simulink model "st"  (R2022b)
settings: Solver=VariableStepAuto  StartTime=0.0  StopTime=1000  RelTol=1e-3
libraries: commsequence2 x2, commdigbbndpm3 x2, dspsrcs4 x2, commfilt2 x2, commchan3 x1, simulink x1, commsink2 x1, commsync2 x1, dspsigops x1
(part 1 of 2)
settings Model: Creator=svdvl  LastModifiedBy=svdvl

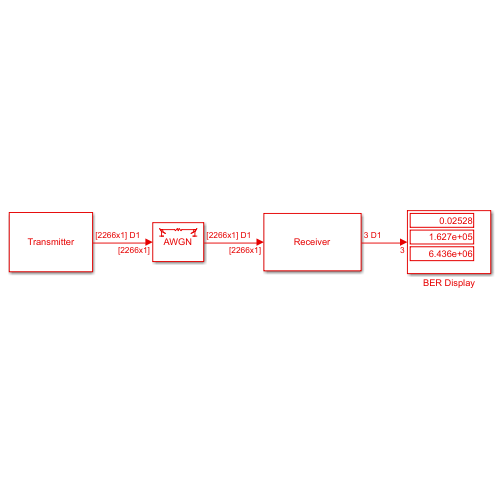
[thumbnail: Simulink's stored preview of the top-level diagram]
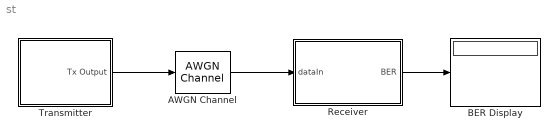
== system st ==
  AWGN Channel : commchan3/AWGN Channel  InputProcessing=Columns as channels (frame based)  seed=1  noiseMode="Signal to noise ratio  (Es/No)"  EbNodB=8  EsNodB=40  SNRdB=8  bitsPerSym=1  Ps=0.5  Tsym=2e-5  variance=1
  BER Display : Display
  Receiver : Subsystem
      mask Display: disp('Receiver')
  Transmitter : Subsystem
      mask Display: disp('Transmitter')
  wires:
  Transmitter/1(Tx Output) -> AWGN Channel/1
  AWGN Channel/1 -> Receiver/1(dataIn)
  Receiver/1(BER) -> BER Display/1

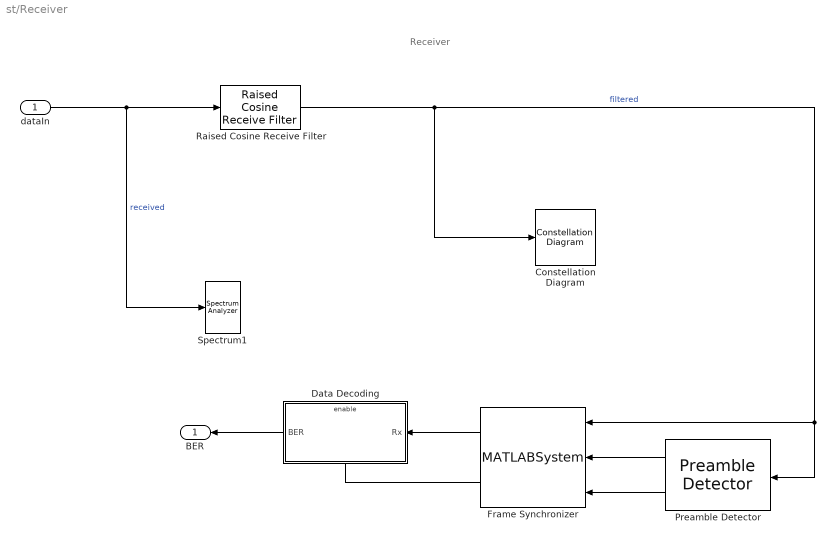
== system st/Receiver ==
  note: Receiver
  dataIn : Inport
  Constellation Diagram : ConstellationDiagram  WindowPosition=[-1346.000000,169.000000,600.000000,600.000000,]  Visible=on  ScopeFrameLocation=window  SamplesPerSymbol=1133  SymbolsToDisplaySource=Property  SymbolsToDisplay=1133  XLimits=[-1.46,1.46]  YLimits=[-1.38,1.38]  DefaultConfigurationName=comm.scopes.ConstellationDiagramBlockCfg
  Data Decoding : Subsystem
      mask Display: disp('Data Decoding');
  Frame Synchronizer : MATLABSystem  System=FrameSynchronizer  Input=Symbol  OutputFrameLength=1133  PreambleLength=13  SimulateUsing=Code generation
      mask Type: FrameSynchronizer
      mask Display:
      | disp(['Frame' char(10) 'Synchronizer']);
      | port_label('input',1,'u');
      | port_label('input',2,'idx');
      | port_label('input',3,'dtMt');
      | port_label('output',1,'Frame');
      | port_label('output',2,'Valid');
  Preamble Detector : commsync2/Preamble Detector  Input=Symbol  Preamble="sqrt(2)/2 * (-1-1i) * ([1     1     1     1     1    -1    -1     1     1    -1     1    -1     1])'"  Threshold=8  DetectionMetricOutput=on  Detections=First  SimulateUsing=Code generation
  Raised Cosine Receive Filter : commfilt2/Raised Cosine Receive Filter  filtType=Square root  R=0.5  filtSpan=12  N=2  downFactor=2  downOffset=0  filterGain=1  InputProcessing=Columns as channels (frame based)  RateOptions=Enforce single-rate processing  framing=Mute  checkCoeff=off  variableName=rcRxFilt  currentFiltSpan=10  D=5  inputOffset=0  sampMode=Mute  saveAsFlag=0  rateMode=Downsampling  checkGain=Normalized  launchFVT=on  roundingMode=Floor  overflowMode=off  coeffDataTypeStr=Inherit: Same word length as input  coeffMin=[]  coeffMax=[]  coeffLastDataTypeStr=Inherit: Same word length as input  accumDataTypeStr=Inherit: Same as product output  accumLastDataTypeStr=Inherit: Same as product output  outputDataTypeStr=Inherit: Same as accumulator  outputMin=[]  outputMax=[]  outputLastDataTypeStr=Inherit: Same as accumulator
  Spectrum1 : SpectrumAnalyzer
  BER : Outport  VectorParamsAs1DForOutWhenUnconnected=off
  wires:
  Raised Cosine Receive Filter/1 -> Constellation Diagram/1, Preamble Detector/1, Frame Synchronizer/1  "filtered"
  dataIn/1 -> Spectrum1/1, Raised Cosine Receive Filter/1  "received"
  Frame Synchronizer/1 -> Data Decoding/1(Rx)
  Preamble Detector/1 -> Frame Synchronizer/2
  Frame Synchronizer/2 -> Data Decoding/Enable
  Data Decoding/1(BER) -> BER/1
  Preamble Detector/2 -> Frame Synchronizer/3

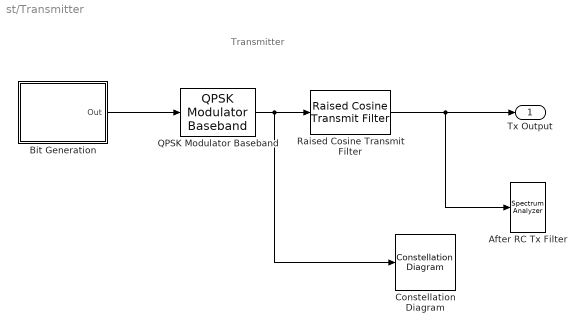
== system st/Transmitter ==
  note: Transmitter
  After RC Tx Filter : SpectrumAnalyzer
  Bit Generation : Subsystem
      mask Display: disp('Bits Generation')
  Constellation Diagram : ConstellationDiagram  WindowPosition=[-1247.000000,248.000000,600.000000,600.000000,]  Visible=on  ScopeFrameLocation=window  DefaultConfigurationName=comm.scopes.ConstellationDiagramBlockCfg
  QPSK Modulator Baseband : commdigbbndpm3/QPSK Modulator Baseband  InType=Bit  Enc=Gray  Ph=pi/4  outDtype=double  outWordLen=16  outUDDataType=sfix(16)  outFracLenMode=Best precision  outFracLen=15  outDataTypeStr=double  outLastDataTypeStr=double
  Raised Cosine Transmit Filter : commfilt2/Raised Cosine Transmit Filter  filtType=Square root  R=0.5  filtSpan=12  N=2  filterGain=1  InputProcessing=Columns as channels (frame based)  RateOptions=Enforce single-rate processing  framing=Mute  checkCoeff=off  variableName=rcTxFilt1  checkGain=Normalized  sampMode=Mute  saveAsFlag=0  currentFiltSpan=10  D=5  launchFVT=on  roundingMode=Floor  overflowMode=off  coeffDataTypeStr=Inherit: Same word length as input  coeffMin=[]  coeffMax=[]  coeffLastDataTypeStr=Inherit: Same word length as input  outputDataTypeStr=Inherit: Same as accumulator  outputMin=[]  outputMax=[]  outputLastDataTypeStr=Inherit: Same as accumulator
  Tx Output : Outport  VectorParamsAs1DForOutWhenUnconnected=off
  wires:
  Raised Cosine Transmit Filter/1 -> Tx Output/1, After RC Tx Filter/1
  Bit Generation/1(Out) -> QPSK Modulator Baseband/1
  QPSK Modulator Baseband/1 -> Constellation Diagram/1, Raised Cosine Transmit Filter/1

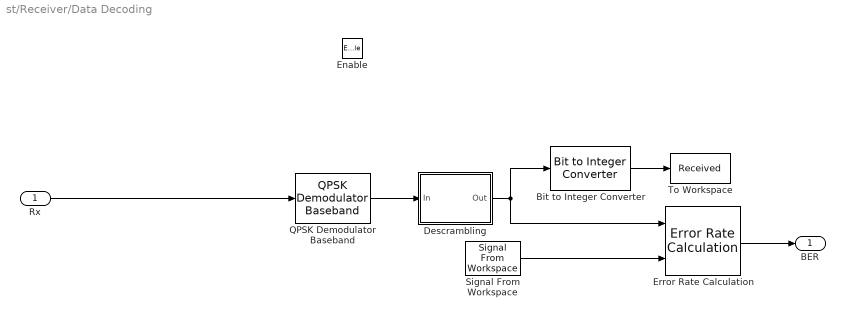
== system st/Receiver/Data Decoding ==
  Rx : Inport
  Enable : EnablePort
  Bit to Integer Converter : simulink/Logic and Bit Operations/Bit to Integer Converter  nbits=7  bitOrder=MSB first  signedOutputValues=Unsigned  outDtype=Inherit via internal rule  outDtypeSigned=Inherit via internal rule
      settings: LibrarySourceBlock=|
      | commutil2/Bit to Integer
      | Converter
  Descrambling : Subsystem
      mask Display: disp('Descrambling');
  Error Rate Calculation : commsink2/Error Rate Calculation  N=0  st_delay=0  cp_mode=Entire frame  subframe=ans.BerMask  PMode=Port  WsName=ErrorVec  RsMode2=off  stop=off  numErr=100  maxBits=1e6
  QPSK Demodulator Baseband : commdigbbndpm3/QPSK Demodulator Baseband  OutType=Bit  DecType=Hard decision  VarSource=Dialog  Variance=1  Dec=Gray  Ph=pi/4  outDtype1=Inherit via internal rule  outDtype2=Inherit via internal rule  derotateFactorWordLen=16  derotateFactorDataTypeStr=Inherit: Same word length as input  derotateFactorLastDataTypeStr=Inherit: Same word length as input
  Signal From Workspace : dspsrcs4/Signal From Workspace  X="[1\t0\t0\t1\t0\t0\t0\t1\t1\t0\t0\t1\t0\t1\t1\t1\t0\t1\t1\t0\t0\t1\t1\t0\t1\t1\t0\t0\t1\t1\t0\t1\t1\t1\t1\t0\t1\t0\t0\t0\t0\t0\t1\t1\t1\t0\t1\t1\t1\t1\t1\t0\t1\t1\t1\t1\t1\t1\t1\t0\t0\t1\t0\t1\t1\t0\t1\t1\t0\t0\t1\t1\t0\t0\t1\t0\t0\t0\t1\t0\t0\t0\t0\t0\t0\t1\t1\t0\t0\t0\t0\t0\t1\t1\t0\t0\t0\t0\t0\t1\t1\t0\t0\t0\t0\t0\t0\t0\t1\t0\t1\t0\t1\t0\t0\t1\t0\t0\t0\t1\t1\t0\t0\t1\t0\t1\t1\t1\t0\t1\t1\t0\t0\t1 ...(+33198 chars)].'"  Ts=1.0116e-05  nsamps=2240  OutputAfterFinalValue=Cyclic repetition  ignoreOrWarnInputAndFrameLengths=on  OutputFrames=off
  To Workspace : ToWorkspace  VariableName=Received  SaveFormat=Structure  SampleTime=-1
      settings: Save2DSignal=2-D array (concatenate along first dimension)
  BER : Outport  VectorParamsAs1DForOutWhenUnconnected=off
  wires:
  Rx/1 -> QPSK Demodulator Baseband/1
  Descrambling/1(Out) -> Error Rate Calculation/1, Bit to Integer Converter/1
  Error Rate Calculation/1 -> BER/1
  QPSK Demodulator Baseband/1 -> Descrambling/1(In)
  Signal From Workspace/1 -> Error Rate Calculation/2
  Bit to Integer Converter/1 -> To Workspace/1
